simulink model "mass_spring_damper"  (R2018b)
settings: Solver=VariableStepAuto  StartTime=0.0  StopTime=10.0  RelTol=1e-3
undefined symbols (not defined in the file): B, F, K, m, x0
settings Model: Creator=student  LastModifiedBy=HP

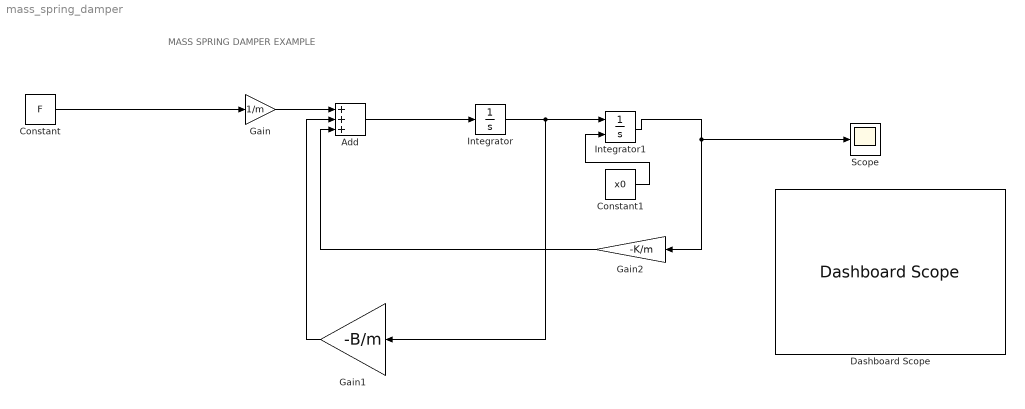
== system mass_spring_damper ==
  note: MASS SPRING DAMPER EXAMPLE
  Add : Sum  Inputs=+++
  Constant : Constant  Value=F
  Constant1 : Constant  Value=x0
  Dashboard Scope : DashboardScope  WebBlockId=13  Ymin=5  Ymax=15
  Gain : Gain  Gain=1/m
  Gain1 : Gain  Gain=-B/m
  Gain2 : Gain  Gain=-K/m
  Integrator : Integrator
  Integrator1 : Integrator  InitialConditionSource=external  InitialCondition=5
  Scope : Scope
  wires:
  Integrator/1 -> Gain1/1, Integrator1/1
  Constant/1 -> Gain/1
  Gain/1 -> Add/1
  Add/1 -> Integrator/1
  Integrator1/1 -> Gain2/1, Scope/1
  Gain2/1 -> Add/3
  Gain1/1 -> Add/2
  Constant1/1 -> Integrator1/2
